simulink model "cc"  (Simulink 7.0)
settings: Solver=ode45  StartTime=0.0  StopTime=inf  FixedStep=0.001  RelTol=1e-3
PostLoadFcn:
  | ,try, rti_mdl_postloadfcn(bdroot, 'UpdateModel', 280, 'rti1005'); catch, disp(lasterr); end,
undefined symbols (not defined in the file or in its folder): none, Rec, SDTV, videoinput
libraries: vipsnks x2, vipfilter x1, vipconversions x1, imaqlib x1, vipanalysis x1
settings Model: Creator=k12_p800a  LastModifiedBy=k12_p800a  BufferReuse=off
settings OptimizationCC: BlockReduction=off  OptimizeBlockIOStorage=off  BufferReuse=off  ExpressionFolding=off  LocalBlockOutputs=off
settings HardwareCC: ProdIntDivRoundTo=Zero  ProdEndianess=BigEndian  ProdHWDeviceType=Specified  TargetIntDivRoundTo=Zero  TargetEndianess=BigEndian
settings RTWCC: SystemTargetFile=rti1005.tlc  MakeCommand=make_rti  TemplateMakefile=rti1005.tmf  Description=dSPACE DS1005 Hardware Platform  ProcessScript=rti1005_make_rtw_hook
settings STFCustomTargetCC: GenFloatMathFcnCalls=ANSI_C  ModelReferenceCompliant=off  MatFileLogging=on  SystemTargetFile=rti1005.tlc
settings GRTTargetCC: ModelReferenceCompliant=off  CompOptLevelCompliant=off  ExtModeMexFile=rti_comm_2
settings CustomProperty: DataType=RTWOptions_EnumType_C__dSPACE_60_matlab_rti1005_tlc_rti1005_InitialSimState  Value=RUN
settings EnumStrPairs: String=RUN

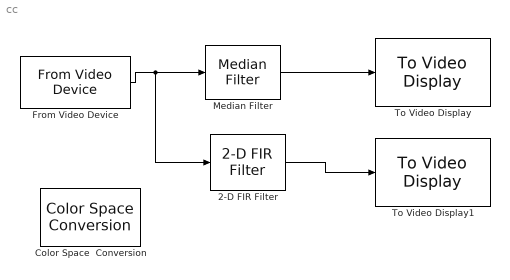
== system cc ==
  2-D FIR Filter : vipfilter/2-D FIR Filter  DialogController=vipDDGCreate  DialogControllerArgs=DataTag0  separable=off  filtSrc=Specify via dialog  filterMtrx=[10 1 10; 10 1 -10; 10 1 10];  verticalFilter=[4 0]  horizontalFilter=[4 0]  outSize=Same as input port I  padType=Constant  padSrc=Specify via dialog  padVal=0  method=Convolution  firstCoeffMode=Specify word length  firstCoeffWordLength=16  firstCoeffFracLength=14  prodOutputMode=Binary point scaling  prodOutputWordLength=32  prodOutputFracLength=10  roundingMode=Floor  overflowMode=off
  Color Space  Conversion : vipconversions/Color Space  Conversion  conversion=Obsolete  conversionActive=R'G'B' to intensity  wp_str=D65  rec=Rec. 601 (SDTV)  sys=1125/60/2:1  imagePorts=One multidimensional signal
  From Video Device : imaqlib/From Video Device  DialogController=imaqcreatedialog  DialogControllerArgs=DataTag2  DeviceMenu=winvideo 1 (WinFast TV2000 XP WDM Video Capture)  Device=winvideo 1 (WinFast TV2000 XP WDM Video Capture)  ObjConstructor=videoinput('winvideo', 1)  VideoFormatMenu=RGB24_720x480  VideoFormat=RGB24_720x480  VideoSource=composite  ROIPosition=[0 0 480 720]  EnableHWTrigger=off  TriggerConfiguration=none/none  SampleTime=1/30  OutputPortsMode=One multidimensional signal  DataType=single  CanDoHWTrigger=no  ReturnedColorSpace=rgb  BlockHandle=4.0026  ROIWidth=720  ROIHeight=480
  Median Filter : vipanalysis/Median Filter  DialogController=vipDDGCreate  DialogControllerArgs=DataTag3  nghbood=[3 3]  outSize=Same as input port I  padType=Constant  padSrc=Specify via dialog  padVal=0  roundingMode=Floor  overflowMode=off
  To Video Display : vipsnks/To Video Display  DialogController=vipDDGCreate  DialogControllerArgs=DataTag4  inputType=Obsolete  imagePorts=One multidimensional signal  OutputDevice=On-screen video monitor  fullScreen=off  videoWindowX=44  videoWindowY=41  saveWindowSize=off  videoWindowWidth=44  videoWindowHeight=41  dataOrg=Column-major
  To Video Display1 : vipsnks/To Video Display  DialogController=vipDDGCreate  DialogControllerArgs=DataTag5  inputType=Obsolete  imagePorts=One multidimensional signal  OutputDevice=On-screen video monitor  fullScreen=off  videoWindowX=44  videoWindowY=41  saveWindowSize=off  videoWindowWidth=44  videoWindowHeight=41  dataOrg=Column-major
  wires:
  From Video Device/1 -> Median Filter/1, 2-D FIR Filter/1
  Median Filter/1 -> To Video Display/1
  2-D FIR Filter/1 -> To Video Display1/1
